simulink model "bicycle_dyn_sim"  (R2020b)
settings: Solver=FixedStepAuto  StartTime=0.0  StopTime=inf  FixedStep=0.01  RelTol=1e-3
libraries: robotlib x8
settings Model: Creator=bascetta  LastModifiedBy=root
settings OptimizationCC: EnhancedBackFolding=on  PassReuseOutputArgsAs=Individual arguments  ZeroExternalMemoryAtStartup=off  ZeroInternalMemoryAtStartup=off  MaxStackSize=64  OptimizeBlockOrder=speed  DifferentSizesBufferReuse=on  OptimizationCustomize=off  EfficientTunableParamExpr=on
settings DebuggingCC: ParameterTunabilityLossMsg=error
settings HardwareCC: ProdBitPerPointer=32  ProdBitPerSizeT=32  ProdBitPerPtrDiffT=32  ProdLargestAtomicFloat=None  ProdIntDivRoundTo=Undefined  ProdEndianess=Unspecified  ProdWordSize=32  ProdHWDeviceType=Generic->Unspecified (assume 32-bit Generic)
settings SFSimCC: MATLABDynamicMemAlloc=off  SimTargetLang=C++
settings RTWCC: Description=Embedded Coder  SystemTargetFile=ert.tlc  HardwareBoard=Robot Operating System (ROS)  TLCOptions="-aInlineSetEventsForThisBaseRateFcn=TLC_FALSE -aSuppressMultiTaskScheduler=TLC_FALSE  -aRateBasedStepFcn=0"  TemplateMakefile=ert_default_tmf  Toolchain=Catkin  TargetLang=C++
settings CodeAppCC: ForceParamTrailComments=on  IgnoreCustomStorageClasses=off  OperatorAnnotations=on  SimulinkDataObjDesc=on  SFDataObjDesc=on  InsertBlockDesc=on
settings ERTTargetCC: SupportContinuousTime=on

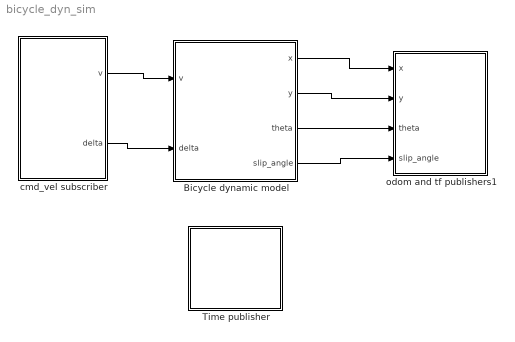
== system bicycle_dyn_sim ==
  Bicycle dynamic model : Subsystem  mask{state0=[88, 182, 0], state1=3.93, RCD=1.6, CFD=1.1, C_f=85000, C_r=70000, m=140, I_z=2500, Linear=1, u=0.65}
      mask prompts: state0 "Initial conditions (x0, y0, beta0)"; state1 "Initial conditions(theta0)"; RCD "Rear-Centre Distance"; CFD "Centre-Front Distance"; C_f "Cornering stiffness front"; C_r "Cornering stiffness rear"; m "Vehicle mass"; I_z "Inertia"; u "Friction"
      mask TypeOptions RCD: Rear-Centre Distance/Value
      mask TypeOptions CFD: Centre-Front Distance/Value
      mask TypeOptions C_f: Cornering stiffness front/Value
      mask TypeOptions C_r: Cornering stiffness rear/Value
      mask TypeOptions m: Vehicle mass/Value
      mask TypeOptions I_z: Inertia/Value
  Time publisher : Subsystem
  cmd_vel subscriber : Subsystem
  odom and tf publishers1 : Subsystem  mask{simPublishRate=100}
      mask prompts: simPublishRate "Publising rate [Hz]"
  wires:
  Bicycle dynamic model/1(x) -> odom and tf publishers1/1(x)
  Bicycle dynamic model/2(y) -> odom and tf publishers1/2(y)
  Bicycle dynamic model/3(theta) -> odom and tf publishers1/3(theta)
  cmd_vel subscriber/1(v) -> Bicycle dynamic model/1(v)
  cmd_vel subscriber/2(delta) -> Bicycle dynamic model/2(delta)
  Bicycle dynamic model/4(slip_angle) -> odom and tf publishers1/4(slip_angle)

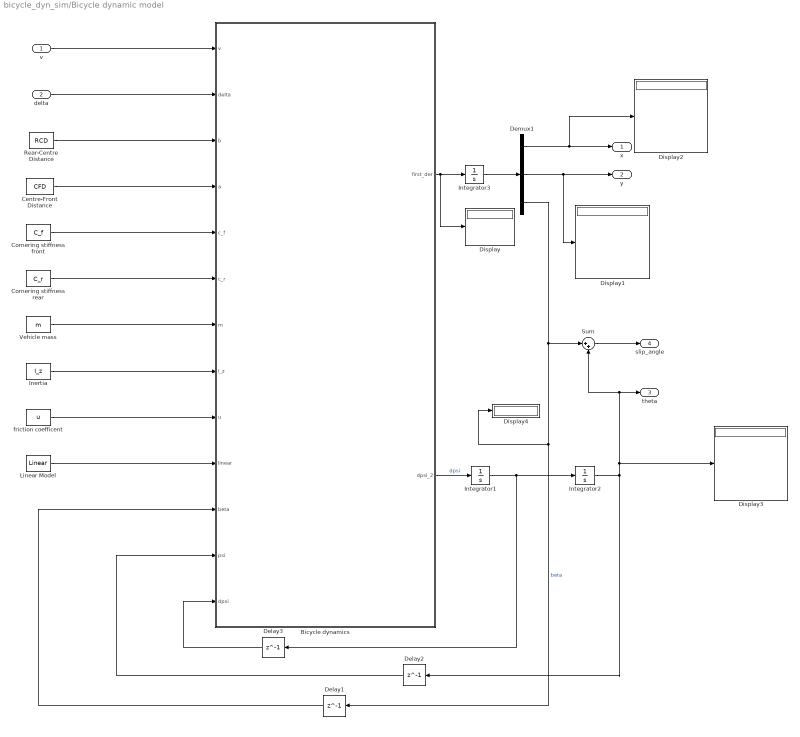
== system bicycle_dyn_sim/Bicycle dynamic model ==
  v : Inport
  delta : Inport  Port=2
  Bicycle dynamics : MATLAB Function  TreatAsAtomicUnit=on
  Centre-Front Distance : Constant  Value=CFD
  Cornering stiffness front : Constant  Value=C_f
  Cornering stiffness rear : Constant  Value=C_r
  Delay1 : Delay  DelayLength=1  InitialCondition=0
  Delay2 : Delay  DelayLength=1  InitialCondition=0
  Delay3 : Delay  DelayLength=1  InitialCondition=0
  Demux1 : Demux  Outputs=3
  Display{,1..4} (5 alike) : Display
  Inertia : Constant  Value=I_z
  Integrator1 : Integrator
  Integrator2 : Integrator  InitialCondition=state1
  Integrator3 : Integrator  InitialCondition=state0
  Linear Model : Constant  Value=Linear
  Rear-Centre Distance : Constant  Value=RCD
  Sum : Sum  Inputs=|++
  Vehicle mass : Constant  Value=m
  friction coefficent : Constant  Value=u
  x : Outport  VectorParamsAs1DForOutWhenUnconnected=off
  y : Outport  Port=2  VectorParamsAs1DForOutWhenUnconnected=off
  theta : Outport  Port=3  VectorParamsAs1DForOutWhenUnconnected=off
  slip_angle : Outport  Port=4  VectorParamsAs1DForOutWhenUnconnected=off
  wires:
  Bicycle dynamics/1(first_der) -> Integrator3/1, Display/1
  Integrator3/1 -> Demux1/1
  Demux1/2 -> y/1, Display1/1
  Demux1/1 -> Display2/1, x/1
  delta/1 -> Bicycle dynamics/2(delta)
  v/1 -> Bicycle dynamics/1(v)
  Rear-Centre Distance/1 -> Bicycle dynamics/3(b)
  Centre-Front Distance/1 -> Bicycle dynamics/4(a)
  Cornering stiffness front/1 -> Bicycle dynamics/5(c_f)
  Cornering stiffness rear/1 -> Bicycle dynamics/6(c_r)
  Vehicle mass/1 -> Bicycle dynamics/7(m)
  Inertia/1 -> Bicycle dynamics/8(i_z)
  Demux1/3 -> Display4/1, Delay1/1, Sum/1  "beta"
  Bicycle dynamics/2(dpsi_2) -> Integrator1/1  "dpsi"
  Sum/1 -> slip_angle/1
  friction coefficent/1 -> Bicycle dynamics/9(u)
  Linear Model/1 -> Bicycle dynamics/10(linear)
  Delay1/1 -> Bicycle dynamics/11(beta)
  Delay2/1 -> Bicycle dynamics/12(psi)
  Delay3/1 -> Bicycle dynamics/13(dpsi)
  Integrator1/1 -> Integrator2/1, Delay3/1
  Integrator2/1 -> Delay2/1, theta/1, Sum/2, Display3/1

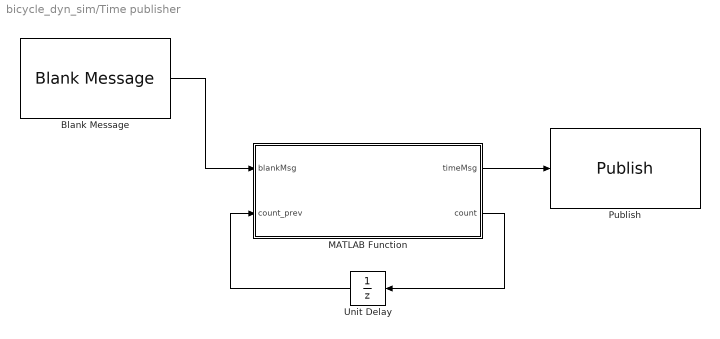
== system bicycle_dyn_sim/Time publisher ==
  Blank Message : robotlib/Blank Message  messageClass=Message  entityType=rosgraph_msgs/Clock  messageType=rosgraph_msgs/Clock  SampleTime=0.01  legacyBusStruct=off
  MATLAB Function : MATLAB Function  TreatAsAtomicUnit=on
  Publish : robotlib/Publish  topicSource=Specify your own  topic=/clock  messageType=rosgraph_msgs/Clock  legacyBusStruct=off  messageQueueLength=1
  Unit Delay : UnitDelay  SampleTime=0.01  HasFrameUpgradeWarning=on
  wires:
  MATLAB Function/1(timeMsg) -> Publish/1
  Blank Message/1 -> MATLAB Function/1(blankMsg)
  MATLAB Function/2(count) -> Unit Delay/1
  Unit Delay/1 -> MATLAB Function/2(count_prev)

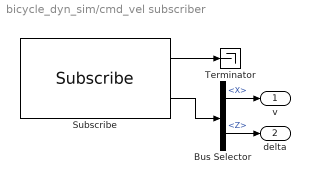
== system bicycle_dyn_sim/cmd_vel subscriber ==
  Bus Selector : BusSelector  OutputSignals=Linear.X,Angular.Z
  Subscribe : robotlib/Subscribe  topicSource=Specify your own  topic=/cmd_vel  messageType=geometry_msgs/Twist  SampleTime=-1  legacyBusStruct=off  messageQueueLength=1
  Terminator : Terminator
  v : Outport
  delta : Outport  Port=2
  wires:
  Bus Selector/1 -> v/1  "<X>"
  Subscribe/2 -> Bus Selector/1
  Subscribe/1 -> Terminator/1
  Bus Selector/2 -> delta/1  "<Z>"

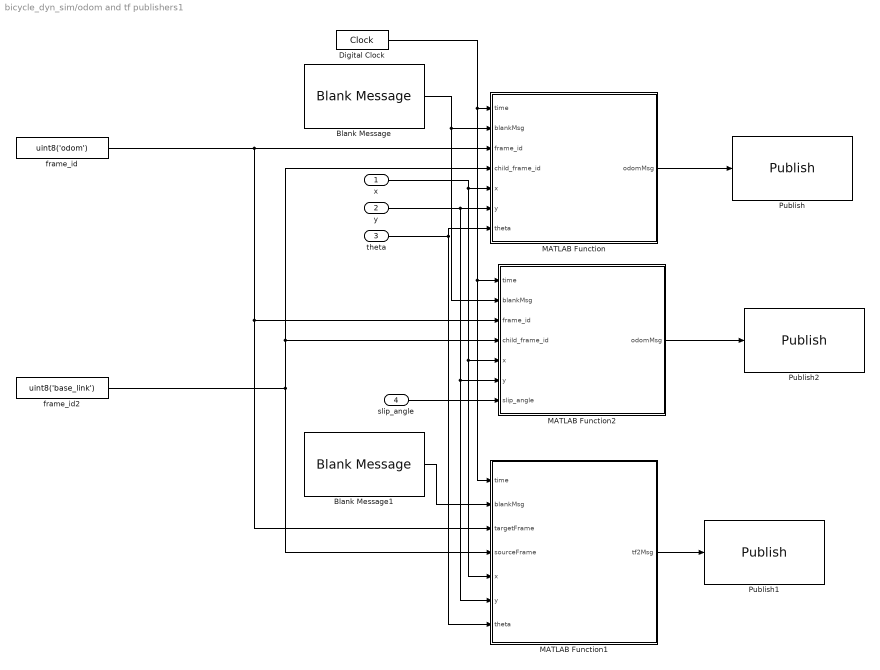
== system bicycle_dyn_sim/odom and tf publishers1 ==
  x : Inport  SampleTime=1/simPublishRate
  y : Inport  Port=2  SampleTime=1/simPublishRate
  theta : Inport  Port=3  SampleTime=1/simPublishRate
  slip_angle : Inport  Port=4  SampleTime=1/simPublishRate
  Blank Message : robotlib/Blank Message  messageClass=Message  entityType=nav_msgs/Odometry  messageType=nav_msgs/Odometry  SampleTime=1/simPublishRate  legacyBusStruct=off
  Blank Message1 : robotlib/Blank Message  messageClass=Message  entityType=tf2_msgs/TFMessage  messageType=tf2_msgs/TFMessage  SampleTime=1/simPublishRate  legacyBusStruct=off
  Digital Clock : DigitalClock  SampleTime=1/simPublishRate
  MATLAB Function : MATLAB Function  TreatAsAtomicUnit=on
  MATLAB Function1 : MATLAB Function  TreatAsAtomicUnit=on
  MATLAB Function2 : MATLAB Function  TreatAsAtomicUnit=on
  Publish : robotlib/Publish  topicSource=Specify your own  topic=/odom  messageType=nav_msgs/Odometry  legacyBusStruct=off  messageQueueLength=1
  Publish1 : robotlib/Publish  topicSource=Specify your own  topic=/tf  messageType=tf2_msgs/TFMessage  legacyBusStruct=off  messageQueueLength=1
  Publish2 : robotlib/Publish  topicSource=Specify your own  topic=/odom_chassis  messageType=nav_msgs/Odometry  legacyBusStruct=off  messageQueueLength=1
  frame_id : Constant  Value=uint8('odom')
  frame_id2 : Constant  Value=uint8('base_link')
  wires:
  theta/1 -> MATLAB Function/7(theta), MATLAB Function1/7(theta)
  y/1 -> MATLAB Function/6(y), MATLAB Function2/6(y), MATLAB Function1/6(y)
  x/1 -> MATLAB Function2/5(x), MATLAB Function1/5(x), MATLAB Function/5(x)
  Blank Message/1 -> MATLAB Function2/2(blankMsg), MATLAB Function/2(blankMsg)
  Digital Clock/1 -> MATLAB Function1/1(time), MATLAB Function2/1(time), MATLAB Function/1(time)
  MATLAB Function1/1(tf2Msg) -> Publish1/1
  Blank Message1/1 -> MATLAB Function1/2(blankMsg)
  frame_id2/1 -> MATLAB Function2/4(child_frame_id), MATLAB Function/4(child_frame_id), MATLAB Function1/4(sourceFrame)
  frame_id/1 -> MATLAB Function1/3(targetFrame), MATLAB Function2/3(frame_id), MATLAB Function/3(frame_id)
  MATLAB Function/1(odomMsg) -> Publish/1
  MATLAB Function2/1(odomMsg) -> Publish2/1
  slip_angle/1 -> MATLAB Function2/7(slip_angle)

== matlab function bicycle_dyn_sim/odom and tf publishers1/MATLAB Function ==
  data: time input; blankMsg input; frame_id input; child_frame_id input; x input; y input; theta input; odomMsg output Bus: SL_Bus_bicycle_dyn_sim_nav_msgs_Odometry
function odomMsg = generate_odom_msg(time,blankMsg,frame_id, child_frame_id,x,y,theta)

% Writing the message header
blankMsg.Header.Stamp.Sec = fix(time);
blankMsg.Header.Stamp.Nsec = fix((time-fix(time))*1e9);
blankMsg.Header.FrameId(1:length(frame_id)) = frame_id;
blankMsg.Header.FrameId_SL_Info.CurrentLength = uint32(length(frame_id));

% Write child frame id "base_link"
blankMsg.ChildFrameId(1:length(child_frame_id)) = child_frame_id;
blankMsg.ChildFrameId_SL_Info.CurrentLength = uint32(length(child_frame_id));
%blankMsg.ChildFrameId = child_frame_id;

% Write pose data
blankMsg.Pose.Pose.Position.X = x;
blankMsg.Pose.Pose.Position.Y = y;
blankMsg.Pose.Pose.Position.Z = 0;

orientation = eul2quat([0, 0, theta], 'ZYX');
blankMsg.Pose.Pose.Orientation.X = orientation(1);
blankMsg.Pose.Pose.Orientation.Y = orientation(2);
blankMsg.Pose.Pose.Orientation.Z = orientation(3);
blankMsg.Pose.Pose.Orientation.W = orientation(4);

odomMsg = blankMsg;

== matlab function bicycle_dyn_sim/Time publisher/MATLAB Function ==
  data: blankMsg input; count_prev input; timeMsg output Bus: SL_Bus_bicycle_dyn_sim_rosgraph_msgs_Clock; count output
function [timeMsg,count] = generate_time_msg(blankMsg,count_prev)

time = count_prev*1e5;

blankMsg.Clock_.Sec = round(time*1e-9);
blankMsg.Clock_.Nsec = round(time-round(time));

count = count_prev+1;

timeMsg = blankMsg;

== matlab function bicycle_dyn_sim/Bicycle dynamic model/Bicycle dynamics ==
  data: v input; delta input; b input; a input; c_f input; c_r input; m input; i_z input; u input; linear input; beta input; psi input; first_der output; dpsi input; dpsi_2 output
function [first_der, dpsi_2] = bicycle_dynamics(v, delta, b, a, c_f, c_r, m, i_z, u,linear, beta ,psi, dpsi)


dx = v*cos(beta + psi);
dy = v*sin(beta + psi);
if(v == 0)
    alpha_f = 0;
    alpha_r = 0;
else
    alpha_f = (beta + ((a*dpsi)/v) - delta );
    alpha_r = (beta - ((b*dpsi)/v));
end

% Normal force
Fz = (m*9.806)/2;

if(linear == 0) % -> linear interaction wheel/surface
    
    if (v == 0) 
        dbeta = 0; 
    else
        dbeta = (1/(m*v))*(-c_f*tan(alpha_f)*cos(delta) - c_r*tan(alpha_r) - m*dpsi*v);
    end
    dpsi_2 = (1/i_z)*(-a*c_f*tan(alpha_f)*cos(delta) + b*c_r*tan(alpha_r));
    
else % -> Non linear
    % front wheel
    if(abs(alpha_f) < atan((3*u*Fz)/c_f)) % -> Full adesion or adhesion/sliding
        Fyf = -c_f*tan(alpha_f) + ((c_f*c_f)/(3*u*Fz))*abs(tan(alpha_f))*tan(alpha_f) - ((c_f*c_f*c_f)/(27*u*Fz*u*Fz))*(tan(alpha_f)*tan(alpha_f)*tan(alpha_f));
    else % -> Full sliding
        Fyf = -u*Fz*sign(alpha_f);
    end
    
    % rear wheel
    if(abs(alpha_r) < atan((3*u*Fz)/c_r)) % -> Full adesion or adhesion/sliding
        Fyr = -c_r*tan(alpha_r) + ((c_r*c_r)/(3*u*Fz))*abs(tan(alpha_r))*tan(alpha_r) - ((c_r*c_r*c_r)/(27*u*Fz*u*Fz))*(tan(alpha_r)*tan(alpha_r)*tan(alpha_r));
    else % -> Full sliding
        Fyr = -u*Fz*sign(alpha_r);
    end
    
    dpsi_2 = (a*Fyf*cos(delta) - b*Fyr)*(1/i_z);
     if (v==0)
         dbeta=0;
    else
         dbeta = (1/(m*v))*(Fyf*cos(delta) + Fyr - m*dpsi*v);
    end 

    
end




first_der = [dx, dy, dbeta];

== matlab function bicycle_dyn_sim/odom and tf publishers1/MATLAB Function1 ==
  data: time input; blankMsg input; targetFrame input; sourceFrame input; x input; y input; tf2Msg output Bus: SL_Bus_bicycle_dyn_sim_tf2_msgs_TFMessage; theta input
function tf2Msg = generate_tf2_msg(time, blankMsg, targetFrame, sourceFrame, x, y, theta)

% Set the number of transforms
blankMsg.Transforms_SL_Info.CurrentLength = uint32(1);


% Writing transform header
% Source frame is "base_link", target frame is "odom" 
blankMsg.Transforms(1).Header.Stamp.Sec = fix(time);
blankMsg.Transforms(1).Header.Stamp.Nsec = fix((time-fix(time))*1e9);
blankMsg.Transforms(1).Header.FrameId(1:length(targetFrame)) = targetFrame;
blankMsg.Transforms(1).Header.FrameId_SL_Info.CurrentLength = uint32(length(targetFrame));
blankMsg.Transforms(1).ChildFrameId(1:length(sourceFrame)) = sourceFrame;
blankMsg.Transforms(1).ChildFrameId_SL_Info.CurrentLength = uint32(length(sourceFrame));

% Writing transform traslation and rotation data
blankMsg.Transforms(1).Transform.Translation.X = x;
blankMsg.Transforms(1).Transform.Translation.Y = y;
blankMsg.Transforms(1).Transform.Translation.Z = 0;

rotation = eul2quat([0, 0, theta], 'ZYX');
blankMsg.Transforms(1).Transform.Rotation.X = rotation(1);
blankMsg.Transforms(1).Transform.Rotation.Y = rotation(2);
blankMsg.Transforms(1).Transform.Rotation.Z = rotation(3);
blankMsg.Transforms(1).Transform.Rotation.W = rotation(4);

tf2Msg = blankMsg;

== matlab function bicycle_dyn_sim/odom and tf publishers1/MATLAB Function2 ==
  data: time input; blankMsg input; frame_id input; child_frame_id input; x input; y input; slip_angle input; odomMsg output Bus: SL_Bus_bicycle_dyn_sim_nav_msgs_Odometry
function odomMsg = generate_odom_msg(time,blankMsg,frame_id, child_frame_id,x,y,slip_angle)

% Writing the message header
blankMsg.Header.Stamp.Sec = fix(time);
blankMsg.Header.Stamp.Nsec = fix((time-fix(time))*1e9);
blankMsg.Header.FrameId(1:length(frame_id)) = frame_id;
blankMsg.Header.FrameId_SL_Info.CurrentLength = uint32(length(frame_id));

% Write child frame id "base_link"
blankMsg.ChildFrameId(1:length(child_frame_id)) = child_frame_id;
blankMsg.ChildFrameId_SL_Info.CurrentLength = uint32(length(child_frame_id));
%blankMsg.ChildFrameId = child_frame_id;

% Write pose data
blankMsg.Pose.Pose.Position.X = x;
blankMsg.Pose.Pose.Position.Y = y;
blankMsg.Pose.Pose.Position.Z = 0;

orientation = eul2quat([0, 0, slip_angle], 'ZYX');
blankMsg.Pose.Pose.Orientation.X = orientation(1);
blankMsg.Pose.Pose.Orientation.Y = orientation(2);
blankMsg.Pose.Pose.Orientation.Z = orientation(3);
blankMsg.Pose.Pose.Orientation.W = orientation(4);

odomMsg = blankMsg;
